simulink model "launcher_dir"  (R2018b)
settings: Solver=ode45  StartTime=0.0  StopTime=10.0  RelTol=1e-3
settings Model: Creator=hlf  LastModifiedBy=12819
settings DataIOCC: SaveFormat=StructureWithTime  ReturnWorkspaceOutputs=on
settings OptimizationCC: LifeSpan=inf
settings DebuggingCC: SFExecutionAtInitializationDiag=none
settings HardwareCC: ProdBitPerSizeT=32  ProdBitPerPtrDiffT=32  ProdWordSize=32  ProdHWDeviceType=Specified
settings CodeAppCC: StateflowObjectComments=on

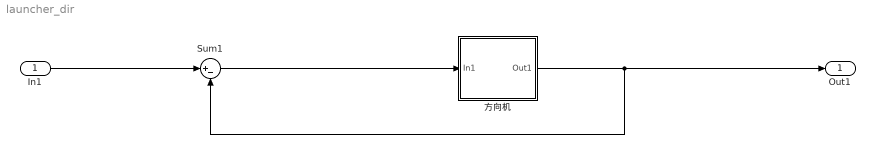
== system launcher_dir ==
  In1 : Inport
  Sum1 : Sum  Inputs=|+-
  方向机 : Subsystem
  Out1 : Outport
  wires:
  方向机/1(Out1) -> Out1/1, Sum1/2
  In1/1 -> Sum1/1
  Sum1/1 -> 方向机/1(In1)

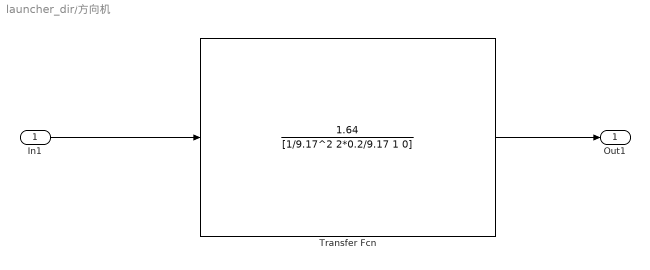
== system launcher_dir/方向机 ==
  In1 : Inport
  Transfer Fcn : TransferFcn  Numerator=[1.64]  Denominator=[1/9.17^2 2*0.2/9.17 1 0]
  Out1 : Outport
  wires:
  Transfer Fcn/1 -> Out1/1
  In1/1 -> Transfer Fcn/1
